simulink model "FCS_Standalone_Model_AADD"  (R2020b)
settings: Solver=VariableStepAuto  StartTime=0.0  StopTime=50  RelTol=1e-3
undefined symbols (not defined in the file or in its folder): Capacity, fuelCellOrg, Internal_resistance, N, Nom_voltage, SOC_initial
libraries: powerlib x8, powerlib_meascontrol x4, simulink x2
settings Model: Creator=oqz0vm8  LastModifiedBy=drim
settings DataIOCC: ReturnWorkspaceOutputs=off
settings DebuggingCC: ArithmeticOperatorsInVariantConditions=warning
settings SFSimCC: SimUseLocalCustomCode=off  CustomCodeUndefinedFunction=UseInterfaceOnly
settings RTWCC: RTWUseLocalCustomCode=off
settings CodeAppCC: StateflowObjectComments=on
settings SimscapeCC: SimscapeNormalizeSystem=off

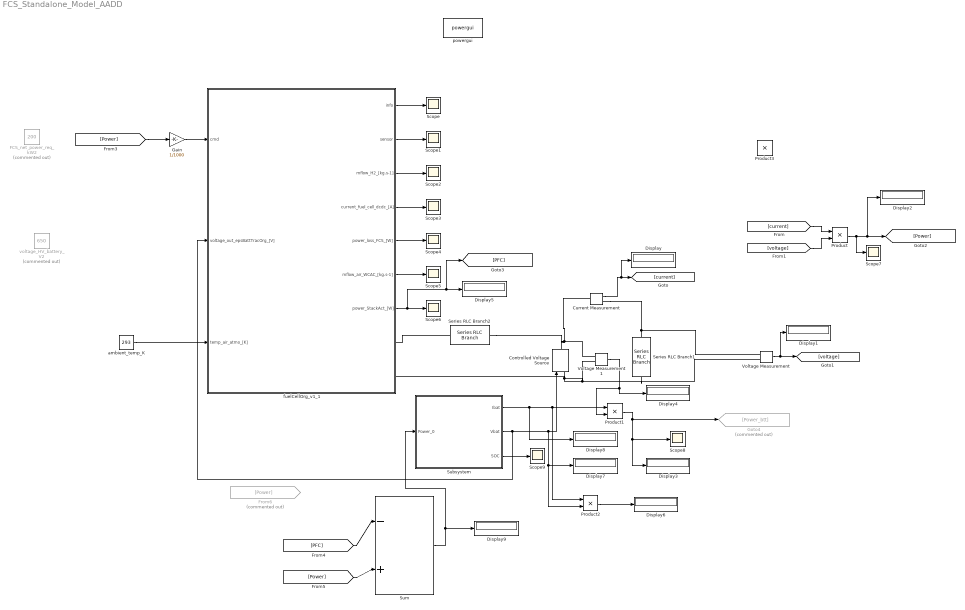
== system FCS_Standalone_Model_AADD ==
  Controlled Voltage Source : powerlib/Electrical Sources/Controlled Voltage Source  Initialize=on  Source_Type=AC  Amplitude=0  Phase=0  Frequency=0  Measurements=None
  Current Measurement : powerlib/Measurements/Current Measurement  PhasorSimulation=off  OutputType=Complex  PSBequivalent=0
  Display{,1..9} (10 alike) : Display
  FCS_net_power_req_kW2 : Constant  Commented=on  Value=200
  From6 : From  Commented=on  GotoTag=Power
  Gain : Gain  Gain=1/1000
  Goto4 : Goto  Commented=on  GotoTag=Power_btt
  Product{,1..3} (4 alike) : Product
  Scope{,1..9} (10 alike) : Scope
  Series RLC Branch1 : powerlib/Elements/Series RLC Branch  LConnTagsString=__new0  RConnTagsString=__new0  BranchType=R  Resistance=0.02  Inductance=1e-3  SetiL0=off  InitialCurrent=0  Capacitance=1e-6  Setx0=off  InitialVoltage=0  Measurements=None
  Series RLC Branch2 : powerlib/Elements/Series RLC Branch  LConnTagsString=__new0  RConnTagsString=__new0  BranchType=R  Resistance=0.0000001  Inductance=1e-3  SetiL0=off  InitialCurrent=0  Capacitance=1e-6  Setx0=off  InitialVoltage=0  Measurements=None
  Subsystem : Subsystem
  Sum : Sum  Inputs=|-+
  Voltage Measurement : powerlib/Measurements/Voltage Measurement  PhasorSimulation=off  OutputType=Complex  PSBequivalent=0
  Voltage Measurement1 : powerlib/Measurements/Voltage Measurement  PhasorSimulation=off  OutputType=Complex  PSBequivalent=0
  ambient_temp_K : Constant  Value=293
  fuelCellOrg_v1_1 : Subsystem
  powergui : powerlib/powergui  Priority=1  SimulationMode=Continuous  SampleTime=50e-6  frequency=60  Iterations=50  frequencyindice=0  Pbase=100e6  ErrMax=1e-4  UnitsV=kV  UnitsW=MW  buscounter=0  FunctionMessages=off  echomessages=off  EnableUseOfTLC=off  CurrentSourceSwitches=off  DisableSnubberDevices=off  DisableRonSwitches=off  DisableVfSwitches=off  DisplayEquations=off  AutomaticDiscreteSolvers=off  SolverType=Tustin/Backward Euler (TBE)  Interpol=off  ExternalGateDelay=off  methode=off  Ts=100  x0status=blocks  SPID=on  SwTol=0  HookPort=off  NonlinearTolerance=1e-4  nMaxIteration=100  ContinueOnMaxIteration=off  RestoreLinks=warning  ResistiveCurrentMeasurement=off  Frange=[0:2:500]  Ylog=off  Xlog=on  ShowGrid=off  save=off  variable=ZData  structure=0  ZoomFFT=off  StartTime=0.0  cycles=1  DisplayStyle=1  fundamental=60  FreqAxis=off  MaxFrequency=1000  frequencyindicesteady=1  RmsSteady=1  display=off
  voltage_HV_battery_V2 : Constant  Commented=on  Value=650
  wires:
  ambient_temp_K/1 -> fuelCellOrg_v1_1/3(temp_air_atmo_[K])
  fuelCellOrg_v1_1/1(info) -> Scope/1
  fuelCellOrg_v1_1/2(sensor) -> Scope1/1
  fuelCellOrg_v1_1/3(mflow_H2_[kg.s-1]) -> Scope2/1
  fuelCellOrg_v1_1/4(current_fuel_cell_dcdc_[A]) -> Scope3/1
  fuelCellOrg_v1_1/5(power_loss_FCS_[W]) -> Scope4/1
  fuelCellOrg_v1_1/6(mflow_air_WCAC_[kg.s-1]) -> Scope5/1
  fuelCellOrg_v1_1/7(power_StackAct_[W]) -> [PFC], Display5/1, Scope6/1
  Voltage Measurement/1 -> Display1/1, [voltage]
  Current Measurement/1 -> Display/1, [current]
  [current] -> Product/1
  [voltage] -> Product/2
  Product/1 -> Scope7/1, Display2/1, [Power]
  Sum/1 -> Subsystem/1(Power_0), Display9/1
  Subsystem/1(Ibat) -> Display8/1, Product2/1, Product1/1
  Subsystem/3(SOC) -> Scope9/1
  Voltage Measurement1/1 -> Display4/1, Product1/2
  Product1/1 -> Goto4/1, Display3/1, Scope8/1
  Product2/1 -> Display6/1
  Subsystem/2(Vbat) -> fuelCellOrg_v1_1/2(voltage_out_epsBattTracOrg_[V]), Display7/1, Product2/2, Controlled Voltage Source/1
  [Power] -> Gain/1
  Gain/1 -> fuelCellOrg_v1_1/1(cmd)
  [Power] -> Sum/2
  [PFC] -> Sum/1
  connections:
  Controlled Voltage Source/LConn1 -- Voltage Measurement1/LConn2 -- Voltage Measurement/LConn2 -- Series RLC Branch1/RConn1 -- fuelCellOrg_v1_1/RConn2
  Current Measurement/LConn1 -- Series RLC Branch2/LConn1 -- Controlled Voltage Source/RConn1 -- Voltage Measurement1/LConn1
  Series RLC Branch1/LConn1 -- Current Measurement/RConn1 -- Voltage Measurement/LConn1
  Series RLC Branch2/RConn1 -- fuelCellOrg_v1_1/RConn1

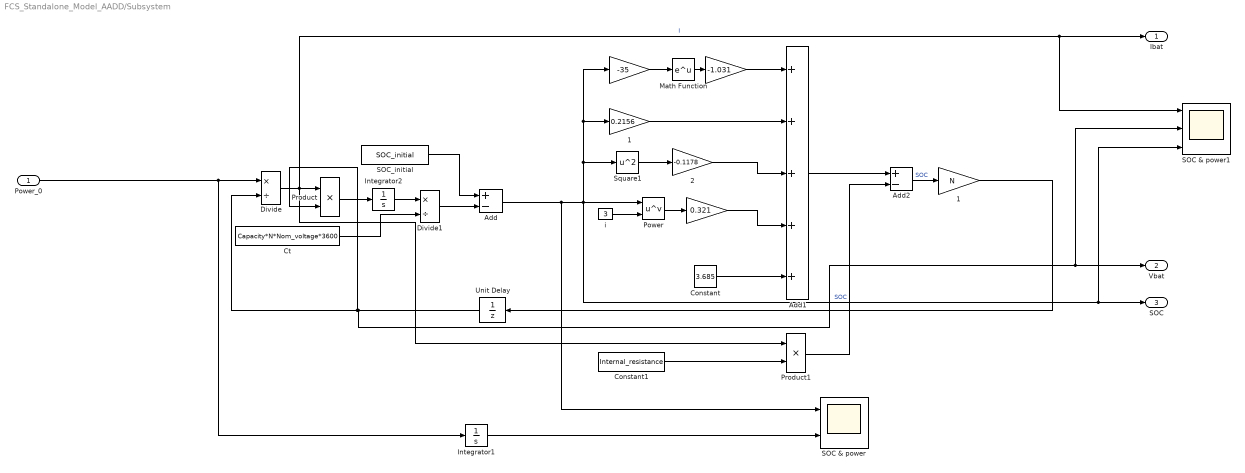
== system FCS_Standalone_Model_AADD/Subsystem ==
  Power_0 : Inport
  " " : Gain  Gain=-1.031
  " " : Gain  Gain=-35
  " " : Gain  Gain=0.321
  " 1" : Gain  Gain=0.2156
  " 1" : Gain  Gain=N
  " 2" : Gain  Gain=-0.1178
  Add : Sum  Inputs=+-
  Add1 : Sum  Inputs=+++++
  Add2 : Sum  Inputs=+-
  Constant : Constant  Value=3.685
  Constant1 : Constant  Value=Internal_resistance
  "Ct " : Constant  Value=Capacity*N*Nom_voltage*3600
  Divide : Product  Inputs=*/
  Divide1 : Product  Inputs=*/
  Integrator1 : Integrator
  Integrator2 : Integrator
  Math Function : Math  SignedPower=on  SaturateOnIntegerOverflow=on
  Power : Math  Operator=pow  SignedPower=on  SaturateOnIntegerOverflow=on
  Product : Product
  Product1 : Product
  SOC & power : Scope  NumInputPorts=2
  SOC & power1 : Scope  NumInputPorts=3
  SOC_initial : Constant  Value=SOC_initial
  Square1 : Math  Operator=square  SignedPower=on  SaturateOnIntegerOverflow=on
  Unit Delay : UnitDelay  InitialCondition=N*Nom_voltage  SampleTime=-1  HasFrameUpgradeWarning=on
  i : Constant  Value=3
  Ibat : Outport  VectorParamsAs1DForOutWhenUnconnected=off
  Vbat : Outport  Port=2  VectorParamsAs1DForOutWhenUnconnected=off
  SOC : Outport  Port=3  VectorParamsAs1DForOutWhenUnconnected=off
  wires:
  " "/1 -> Add1/1
  Integrator2/1 -> Divide1/1
  i/1 -> Power/2
  " 1"/1 -> Add1/2
  Divide/1 -> Ibat/1, SOC & power1/1, Product1/1, Product/1  "I"
  Square1/1 -> " 2"/1
  Add2/1 -> " 1"/1  "SOC"
  Power_0/1 -> Integrator1/1, Divide/1
  " 1"/1 -> Unit Delay/1
  Add/1 -> SOC & power/1, SOC/1, SOC & power1/3, Power/1, " 1"/1, " "/1, Square1/1  "SOC"
  Integrator1/1 -> SOC & power/2
  Constant1/1 -> Product1/2
  Unit Delay/1 -> Vbat/1, SOC & power1/2, Product/2, Divide/2
  "Ct "/1 -> Divide1/2
  Power/1 -> " "/1
  Divide1/1 -> Add/2
  " 2"/1 -> Add1/3
  SOC_initial/1 -> Add/1
  Constant/1 -> Add1/5
  " "/1 -> Math Function/1
  " "/1 -> Add1/4
  Add1/1 -> Add2/1
  Product/1 -> Integrator2/1
  Product1/1 -> Add2/2
  Math Function/1 -> " "/1

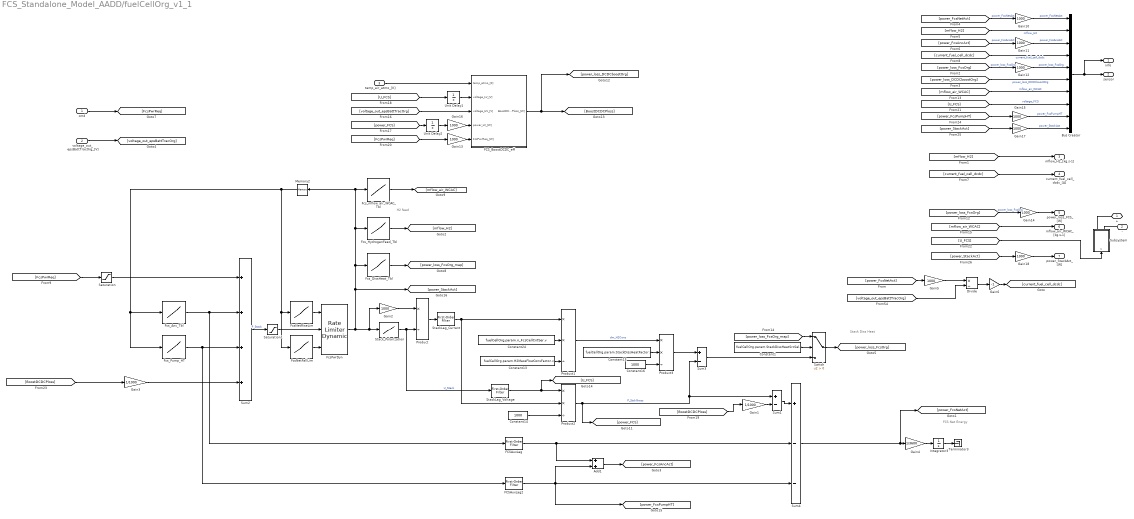
== system FCS_Standalone_Model_AADD/fuelCellOrg_v1_1 ==
  note: FCS Net Energy
  note: Stack Diss Heat
  note: H2 feed
  cmd : Inport
  voltage_out_epsBattTracOrg_[V] : Inport  Port=2
  temp_air_atmo_[K] : Inport  Port=3
  Add1 : Sum
  Bus Creator : BusCreator  Inputs=10
  Constant1 : Constant  Value=fuelCellOrg.param.StackDissHeatSrcSel.v
  Constant13 : Constant  Value=fuelCellOrg.param.H2MassFlowConsFactor.v
  Constant14 : Constant  Value=1000
  Constant15 : Constant  Value=fuelCellOrg.param.StackDissHeatFactor.v
  Constant16 : Constant  Value=1000
  Constant24 : Constant  Value=fuelCellOrg.param.n_FcsCellCntSer.v
  Divide : Product  Inputs=*/
  FCSAuxLag : powerlib_meascontrol/Filters/First-Order Filter  FilterType=Lowpass  Tc=fuelCellOrg.param.t_FcsAncLag.v  Ts=0  Initialize=on  Vac_Init=[0, 0, 60]  Vdc_Init=0  PlotResponse=off  FreqRange="[0,  200,  1]"
  FCSAuxLag2 : powerlib_meascontrol/Filters/First-Order Filter  FilterType=Lowpass  Tc=fuelCellOrg.param.t_FcsAncLag.v  Ts=0  Initialize=on  Vac_Init=[0, 0, 60]  Vdc_Init=0  PlotResponse=off  FreqRange="[0,  200,  1]"
  FCS_BoostDCDC_eff : Subsystem
  FcsNetFallLim : Lookup_n-D  NumberOfTableDimensions=1  BreakpointsForDimension1=fuelCellOrg.param.FcsNetFallLim.x  Table=fuelCellOrg.param.FcsNetFallLim.v  ExtrapMethod=Clip  UseLastTableValue=on  InternalRulePriority=Speed  RndMeth=Simplest  InputSameDT=on
  FcsNetRiseLim : Lookup_n-D  NumberOfTableDimensions=1  BreakpointsForDimension1=fuelCellOrg.param.FcsNetRiseLim.x  Table=fuelCellOrg.param.FcsNetRiseLim.v  ExtrapMethod=Clip  UseLastTableValue=on  InternalRulePriority=Speed  RndMeth=Simplest  InputSameDT=on
  FcsPwrDyn : simulink/Discontinuities/Rate Limiter Dynamic
  Fcs_Anc_Tbl : Lookup_n-D  NumberOfTableDimensions=1  BreakpointsForDimension1=fuelCellOrg.param.Fcs_Anc_Tbl.x  Table=fuelCellOrg.param.Fcs_Anc_Tbl.v  ExtrapMethod=Clip  UseLastTableValue=on  InternalRulePriority=Speed  RndMeth=Simplest  InputSameDT=on
  Fcs_DissHeat_Tbl : Lookup_n-D  NumberOfTableDimensions=1  BreakpointsForDimension1=fuelCellOrg.param.Fcs_DissHeat_Tbl.x  Table=fuelCellOrg.param.Fcs_DissHeat_Tbl.v  ExtrapMethod=Clip  UseLastTableValue=on  InternalRulePriority=Speed  RndMeth=Simplest  InputSameDT=on
  Fcs_HydrogenFeed_Tbl : Lookup_n-D  NumberOfTableDimensions=1  BreakpointsForDimension1=fuelCellOrg.param.Fcs_HydrogenFeed_Tbl.x  Table=fuelCellOrg.param.Fcs_HydrogenFeed_Tbl.v  ExtrapMethod=Clip  UseLastTableValue=on  InternalRulePriority=Speed  RndMeth=Simplest  InputSameDT=on
  Fcs_Pump_HT : Lookup_n-D  NumberOfTableDimensions=1  BreakpointsForDimension1=fuelCellOrg.param.P_FcsPumpHT.x  Table=fuelCellOrg.param.P_FcsPumpHT.v  ExtrapMethod=Clip  UseLastTableValue=on  InternalRulePriority=Speed  RndMeth=Simplest  InputSameDT=on
  Fcs_mflow_air_WCAC_Tbl : Lookup_n-D  NumberOfTableDimensions=1  BreakpointsForDimension1=fuelCellOrg.param.Fcs_mflow_air_WCAC_Tbl.x  Table=fuelCellOrg.param.Fcs_mflow_air_WCAC_Tbl.v  ExtrapMethod=Clip  UseLastTableValue=on  InternalRulePriority=Speed  RndMeth=Simplest  InputSameDT=on
  Gain1 : Gain  Gain=1/1000
  Gain{2,5,10..18} (11 alike) : Gain  Gain=1000
  Gain3 : Gain  Gain=1/1000
  Gain4 : Gain  Gain=1/3600
  Gain6 : Gain  Gain=-1
  Integrator3 : Integrator
  Memory2 : Memory
  Product : Product  Inputs=*/
  Product1 : Product  Inputs=**/
  Product2 : Product  Inputs=**/
  Product3 : Product  Inputs=**/
  Saturation : Saturate  UpperLimit=fuelCellOrg.param.P_FcsNetMaxLim.v  LowerLimit=0
  Saturation1 : Saturate  UpperLimit=max(fuelCellOrg.param.Fcs_Anc_Tbl.x)  LowerLimit=0
  StackLag_Current : powerlib_meascontrol/Filters/First-Order Filter  FilterType=Lowpass  Tc=fuelCellOrg.param.t_StckCurrLag.v  Ts=0  Initialize=on  Vac_Init=[0, 0, 60]  Vdc_Init=0  PlotResponse=off  FreqRange="[0,  200,  1]"
  StackLag_Voltage : powerlib_meascontrol/Filters/First-Order Filter  FilterType=Lowpass  Tc=fuelCellOrg.param.t_StckVoltLag.v  Ts=0  Initialize=on  Vac_Init=[0, 0, 60]  Vdc_Init=0  PlotResponse=off  FreqRange="[0,  200,  1]"
  Stack_Polarization : Lookup  InputValues=fuelCellOrg.param.StackPolarization.x  Table=fuelCellOrg.param.StackPolarization.v  LookUpMeth=Interpolation-Use End Values
  Subsystem : Subsystem
  Sum1 : Sum  Inputs=+-
  Sum2 : Sum  Inputs=++++
  Sum3 : Sum  Inputs=+-
  Sum4 : Sum  Inputs=+--
  Switch : Switch  Criteria=u2 > Threshold
  Terminator3 : Terminator
  Unit Delay1 : UnitDelay  SampleTime=-1  HasFrameUpgradeWarning=on
  Unit Delay2 : UnitDelay  SampleTime=-1  HasFrameUpgradeWarning=on
  + : PMIOPort  Side=Right
  - : PMIOPort  Port=2  Side=Right
  info : Outport
  sensor : Outport  Port=2
  mflow_H2_[kg.s-1] : Outport  Port=3
  current_fuel_cell_dcdc_[A] : Outport  Port=4
  power_loss_FCS_[W] : Outport  Port=5
  mflow_air_WCAC_[kg.s-1] : Outport  Port=6
  power_StackAct_[W] : Outport  Port=7
  wires:
  Saturation1/1 -> FcsPwrDyn/2
  Fcs_Pump_HT/1 -> Sum2/3, FCSAuxLag2/1
  FCSAuxLag2/1 -> Sum4/3, Add1/2, [power_FcsPumpHT]
  Constant15/1 -> Product3/2
  Add1/1 -> [power_FcsAncAct]
  Gain3/1 -> Sum2/4
  [mflow_H2] -> mflow_H2_[kg.s-1]/1
  Gain17/1 -> Bus Creator/10  "power_StackAct"
  Gain18/1 -> power_StackAct_[W]/1
  Fcs_DissHeat_Tbl/1 -> [power_loss_FcsOrg_map]
  Gain1/1 -> Sum1/2
  Memory2/1 -> FcsNetRiseLim/1, FcsNetFallLim/1, Fcs_Pump_HT/1, Fcs_Anc_Tbl/1
  FcsNetFallLim/1 -> FcsPwrDyn/3
  Gain15/1 -> Bus Creator/9  "power_FcsPumpHT"
  Fcs_mflow_air_WCAC_Tbl/1 -> [mflow_air_WCAC]
  FcsNetRiseLim/1 -> FcsPwrDyn/1
  Product3/1 -> Sum3/1
  FcsPwrDyn/1 -> Stack_Polarization/1, Gain2/1, [power_StackAct], Fcs_HydrogenFeed_Tbl/1, Memory2/1, Fcs_mflow_air_WCAC_Tbl/1, Fcs_DissHeat_Tbl/1
  Switch/1 -> [power_loss_FcsOrg]
  Gain13/1 -> FCS_BoostDCDC_eff/5(FcsPwrReq_[W])
  [BoostDCDCPloss] -> Gain3/1
  [mflow_air_WCAC] -> mflow_air_WCAC_[kg.s-1]/1
  Product1/1 -> Product3/1  "dm_H2Cons"
  Gain4/1 -> Integrator3/1
  Constant24/1 -> Product1/2
  StackLag_Voltage/1 -> Product2/1, [U_FCS]
  Constant13/1 -> Product1/3
  [power_StackAct] -> Gain17/1
  Bus Creator/1 -> sensor/1, info/1
  [power_FcsNetAct] -> Gain10/1  "power_FcsNetAct"
  [BoostDCDCPloss] -> Gain1/1
  [power_loss_FcsOrg_map] -> Switch/1
  Saturation/1 -> Sum2/1
  Product2/1 -> [power_FCS], Sum3/2, Sum1/1  "P_StckGross"
  Fcs_HydrogenFeed_Tbl/1 -> [mflow_H2]
  Sum4/1 -> Gain4/1, [power_FcsNetAct]
  Constant14/1 -> Product2/3
  StackLag_Current/1 -> Product1/1, Product2/2
  Constant1/1 -> Switch/2
  Sum2/1 -> Saturation1/1  "P_Stack"
  [power_StackAct] -> Gain18/1
  [mflow_air_WCAC] -> Bus Creator/7  "mflow_air_WCAC"
  [FcsPwrReq] -> Gain13/1
  [power_FcsPumpHT] -> Gain15/1
  Integrator3/1 -> Terminator3/1
  [U_FCS] -> Bus Creator/8  "voltage_FCS"
  FCSAuxLag/1 -> Sum4/2, Add1/1
  [FcsPwrReq] -> Saturation/1
  Product/1 -> StackLag_Current/1
  Gain2/1 -> Product/1
  Sum1/1 -> Sum4/1
  Constant16/1 -> Product3/3
  Stack_Polarization/1 -> StackLag_Voltage/1, Product/2  "U_Stack"
  [power_FcsAncAct] -> Gain11/1  "power_FcsAncAct"
  [U_FCS] -> Unit Delay1/1
  [power_loss_DCDCboostOrg] -> Bus Creator/6  "power_loss_DCDCboostOrg"
  Divide/1 -> Gain6/1
  [current_fuel_cell_dcdc] -> current_fuel_cell_dcdc_[A]/1
  [voltage_out_epsBattTracOrg] -> FCS_BoostDCDC_eff/3(voltage_HV_[V])
  Unit Delay2/1 -> Gain16/1
  [power_FCS] -> Unit Delay2/1
  [mflow_H2] -> Bus Creator/2  "mflow_H2"
  Gain5/1 -> Divide/1
  Sum3/1 -> Switch/3
  FCS_BoostDCDC_eff/1(BoostDCDCPloss_[W]) -> [BoostDCDCPloss], [power_loss_DCDCboostOrg]
  Gain6/1 -> [current_fuel_cell_dcdc]
  Gain10/1 -> Bus Creator/1  "power_FcsNetAct"
  Gain16/1 -> FCS_BoostDCDC_eff/4(power_LV_[W])
  voltage_out_epsBattTracOrg_[V]/1 -> [voltage_out_epsBattTracOrg]
  [power_FcsNetAct] -> Gain5/1
  Fcs_Anc_Tbl/1 -> FCSAuxLag/1, Sum2/2
  Gain11/1 -> Bus Creator/3  "power_FcsAncAct"
  Gain14/1 -> power_loss_FCS_[W]/1
  [voltage_out_epsBattTracOrg] -> Divide/2
  Gain12/1 -> Bus Creator/5  "power_loss_FcsOrg"
  [current_fuel_cell_dcdc] -> Bus Creator/4  "current_fuel_cell_dcdc"
  Unit Delay1/1 -> FCS_BoostDCDC_eff/2(voltage_LV_[V])
  temp_air_atmo_[K]/1 -> FCS_BoostDCDC_eff/1(temp_atmo_[K])
  [power_loss_FcsOrg] -> Gain12/1  "power_loss_FcsOrg"
  cmd/1 -> [FcsPwrReq]
  [power_loss_FcsOrg] -> Gain14/1  "power_loss_FcsOrg"
  [U_FCS] -> Subsystem/1(s)
  connections:
  +/RConn1 -- Subsystem/RConn1
  -/RConn1 -- Subsystem/RConn2

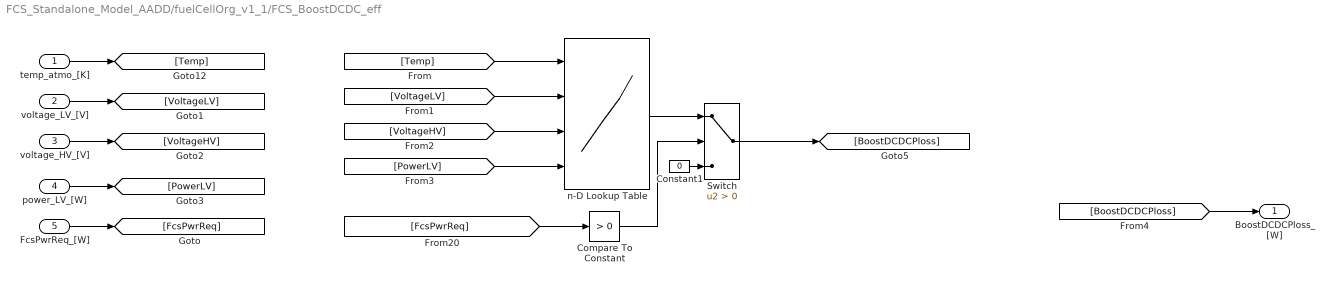
== system FCS_Standalone_Model_AADD/fuelCellOrg_v1_1/FCS_BoostDCDC_eff ==
  temp_atmo_[K] : Inport
  voltage_LV_[V] : Inport  Port=2
  voltage_HV_[V] : Inport  Port=3
  power_LV_[W] : Inport  Port=4
  FcsPwrReq_[W] : Inport  Port=5
  Compare To Constant : simulink/Logic and Bit Operations/Compare To Constant  relop=>  const=0  OutDataTypeStr=boolean
  Constant1 : Constant  Value=0
  Switch : Switch  Criteria=u2 > Threshold
  n-D Lookup Table : Lookup_n-D  NumberOfTableDimensions=4  BreakpointsForDimension1=fuelCellOrg.param.eta_DcDcBoostMap4d.Temp  BreakpointsForDimension2=fuelCellOrg.param.eta_DcDcBoostMap4d.VoltageLV  BreakpointsForDimension3=fuelCellOrg.param.eta_DcDcBoostMap4d.VoltageHV  BreakpointsForDimension4=fuelCellOrg.param.eta_DcDcBoostMap4d.PowerLV  Table=fuelCellOrg.param.eta_DcDcBoostMap4d.v  InternalRulePriority=Speed  RndMeth=Simplest  InputSameDT=on
      settings: InputPortMap=u0,u1,u2,u3
  BoostDCDCPloss_[W] : Outport
  wires:
  FcsPwrReq_[W]/1 -> [FcsPwrReq]
  [FcsPwrReq] -> Compare To Constant/1
  Switch/1 -> [BoostDCDCPloss]
  [BoostDCDCPloss] -> BoostDCDCPloss_[W]/1
  [VoltageLV] -> n-D Lookup Table/2
  [Temp] -> n-D Lookup Table/1
  power_LV_[W]/1 -> [PowerLV]
  voltage_HV_[V]/1 -> [VoltageHV]
  voltage_LV_[V]/1 -> [VoltageLV]
  temp_atmo_[K]/1 -> [Temp]
  n-D Lookup Table/1 -> Switch/1
  [VoltageHV] -> n-D Lookup Table/3
  Constant1/1 -> Switch/3
  Compare To Constant/1 -> Switch/2
  [PowerLV] -> n-D Lookup Table/4

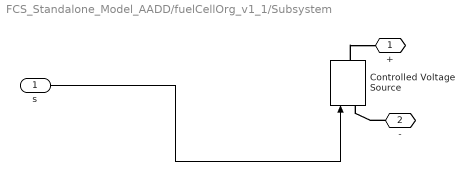
== system FCS_Standalone_Model_AADD/fuelCellOrg_v1_1/Subsystem ==
  s : Inport
  Controlled Voltage Source : powerlib/Electrical Sources/Controlled Voltage Source  Initialize=on  Source_Type=DC  Amplitude=0  Phase=0  Frequency=0  Measurements=None
  + : PMIOPort  Side=Right
  - : PMIOPort  Port=2  Side=Right
  wires:
  s/1 -> Controlled Voltage Source/1
  connections:
  -/RConn1 -- Controlled Voltage Source/LConn1
  Controlled Voltage Source/RConn1 -- +/RConn1
